simulink model "multirate_d4_cauer2_pc_tmp"  (Simulink 7.8)
settings: Solver=FixedStepDiscrete  SolverMode=SingleTasking  StartTime=0.0  StopTime=5.0  RelTol=1e-3
undefined symbols (not defined in the file or in its folder): a, b
libraries: dspsigops x2, dspwin32 x2
settings Model: Creator=Wirnitzer  LastModifiedBy=Wirnitzer
settings DataIOCC: LimitDataPoints=off
settings OptimizationCC: BooleanDataType=off  OptimizeModelRefInitCode=on  LifeSpan=1
settings DebuggingCC: SaveWithParameterizedLinksMsg=none  SignalResolutionControl=TryResolveAllWithWarning  SolverPrmCheckMsg=none  MultiTaskDSMMsg=warning  MultiTaskCondExecSysMsg=none  StrictBusMsg=None
settings HardwareCC: TargetUnknown=on
settings RTWCC: SystemTargetFile=ert.tlc  GenCodeOnly=on  TemplateMakefile=ert_default_tmf  ProcessScript=ert_make_rtw_hook  IncludeERTFirstTime=on
settings CodeAppCC: IgnoreCustomStorageClasses=off
settings ERTTargetCC: MultiwordLength=2048  GenerateSampleERTMain=on  ERTCustomFileTemplate=example_file_process.tlc  ConvertIfToSwitch=off  SuppressUnreachableDefaultCases=off

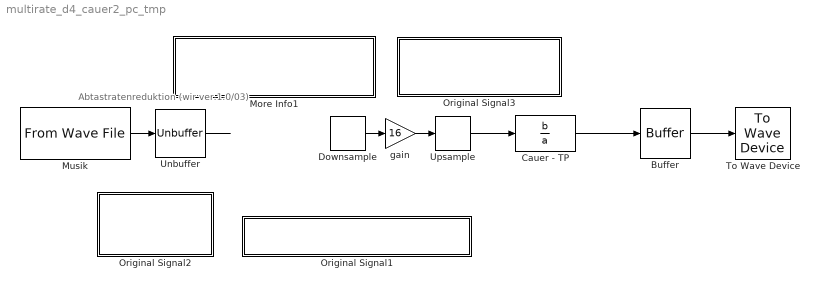
== system multirate_d4_cauer2_pc_tmp ==
  note: Abtastratenreduktion
      | (wir ver.1.0/03)
  " Cauer - TP " : DiscreteFilter  Numerator=b  Denominator=a
  Buffer : Buffer  N=256
  Downsample : dspsigops/Downsample  N=4  phase=0  InputProcessing=Inherited (this choice will be removed - see release notes)  RateOptions=Enforce single-rate processing  smode=Allow multirate  fmode=Maintain input frame size  ic=0
  More Info1 : Subsystem
      mask Display: disp(' Aufgaben')
  Musik : dspwin32/From Wave File  FileName=speech_dft  SamplesPerFrame=256  MinBufSize=256  dType=double  bLoop=off  timesToPlay=1  restartMode=immediately after last sample  firstSampleOutput=off  lastSampleOutput=off
  Original Signal1 : Subsystem  Description=Filterentwurf übernehmen
      settings: OpenFcn=[b,a] = filtdemo('getfilt')
      mask Type: Cauer-Filter
      mask Display: disp('Momentanen Entwurf übernehmen')
  Original Signal2 : Subsystem  Description=Filterentwurf
      settings: OpenFcn=filtdemo
      mask Type: Cauer-Filter
      mask Display: disp('Filterentwurf')
  Original Signal3 : Subsystem  Description=Initialisierung Cauer-Filter
      settings: OpenFcn="b = [    0.0237    0.0129    0.0129    0.0237] ; a = [  1.0000   -2.2668    2.0908   -0.7508];"
      mask Type: Cauer-Filter
      mask Display: disp('Init default Cauer-Filter')
  To Wave Device : dspwin32/To Wave Device  bufDuration=2  determineBufSize=on  userIntBufSize=256  initDelay=0.1  useDefaultDevice=on  userDeviceID=Microsoft RDP Audio Driver  enable24Bit=off
  Unbuffer : Unbuffer
  Upsample : dspsigops/Upsample  N=4  phase=0  InputProcessing=Inherited (this choice will be removed - see release notes)  RateOptions=Allow multirate processing  ic=0  mode=Unused parameter value
  gain : Gain  Gain=16  SaturateOnIntegerOverflow=on  OutDataTypeStr=Inherit: Same as input  ParamDataTypeStr=Inherit: Same as input
  wires:
  ? -> ?
  gain/1 -> Upsample/1
  " Cauer - TP "/1 -> Buffer/1
  ? -> Downsample/1
  Musik/1 -> Unbuffer/1
  Unbuffer/1 -> ?
  Downsample/1 -> gain/1
  Upsample/1 -> " Cauer - TP "/1
  Buffer/1 -> To Wave Device/1

== system multirate_d4_cauer2_pc_tmp/More Info1 ==
  note: Abtastratenreduktion
      | (B.Wir 23.5.03 ver  0.1)
      |
      | Cauer-Filter sind für die Audioverarbeitung besonders geeignet, da sie eine hohe
      | Flankensteilheit bei geringer Filterordnung ermöglichen.
      | Die nichtlineare Phase der Cauer-Filter ist wegen dee Phasentaubheit des Gehörs unwesentlich.
      |
      | Mit den Feld 'Filterentwurf' können Sie unterschiedliche Filterentwurfmethoden testen.
      | Die Übernahme der Filterkoeffizienten erfolgt bei geöffneten Entwurfsfenster!
      |
      |
      | Aufgaben:
      |
      | 0) Doppelklick auf das Feld 'Default Cauer-Filter' initialisiert die beiden grünen  Cauer-Tiefpässe.
      |     Starten Sie die Simulation!
      |     Starten Sie den Filterentwurf. Welche Grenzfrequenz und welche Sperrdämfung sind sinnvoll?
      |     Schätzen Sie den Rechenzeitbedarf bei einem  Elliptischen (Cauer-), Fenster- und REMEZ-Entwurf ab!
      |
      | 1) Entfernen Sie den grünen Cauer-Tiefpass am Ausgang und starten Sie die Simulation. Erklären Sie
      |     die Störungen indem Sie den Betrag des Signalspektrumdurch entlang der Signalkette skizzieren.
      |
      | 2) Entfernen Sie nun zusätzlich den  Cauer-Tiefpass am Eingang und erklären Sie die Störungen.
      |
      | 3) Entfernen Sie nur den  Cauer-Tiefpass am Eingang und erklären Sie die Störungen.

== system multirate_d4_cauer2_pc_tmp/Original Signal1 ==

== system multirate_d4_cauer2_pc_tmp/Original Signal2 ==

== system multirate_d4_cauer2_pc_tmp/Original Signal3 ==
